simulink model "new_model"  (R2023a)
(part 4 of 4)

  Bus Selector:RadarSensor:4_OBJ_RCS_BS/5 -> RadarSensor:4.OBJ_RCS_5/1  "<OBJ_RCS_5>"
  Bus Selector:RadarSensor:4_OBJ_RCS_BS/6 -> RadarSensor:4.OBJ_RCS_6/1  "<OBJ_RCS_6>"
  Bus Selector:RadarSensor:4_OBJ_RCS_BS/7 -> RadarSensor:4.OBJ_RCS_7/1  "<OBJ_RCS_7>"
  Bus Selector:RadarSensor:4_OBJ_RCS_BS/8 -> RadarSensor:4.OBJ_RCS_8/1  "<OBJ_RCS_8>"
  Bus Selector:RadarSensor:4_OBJ_RCS_BS/9 -> RadarSensor:4.OBJ_RCS_9/1  "<OBJ_RCS_9>"
  Bus Selector:RadarSensor:4_OBJ_RCS_BS/10 -> RadarSensor:4.OBJ_RCS_10/1  "<OBJ_RCS_10>"
  Bus Selector:RadarSensor:4_OBJ_RCS_BS/11 -> RadarSensor:4.OBJ_RCS_11/1  "<OBJ_RCS_11>"
  Bus Selector:RadarSensor:4_OBJ_RCS_BS/12 -> RadarSensor:4.OBJ_RCS_12/1  "<OBJ_RCS_12>"
  Bus Selector:RadarSensor:4_OBJ_RCS_BS/13 -> RadarSensor:4.OBJ_RCS_13/1  "<OBJ_RCS_13>"
  Bus Selector:RadarSensor:4_OBJ_RCS_BS/14 -> RadarSensor:4.OBJ_RCS_14/1  "<OBJ_RCS_14>"
  Bus Selector:RadarSensor:4_OBJ_RCS_BS/15 -> RadarSensor:4.OBJ_RCS_15/1  "<OBJ_RCS_15>"
  Bus Selector:RadarSensor:4_OBJ_RCS_BS/16 -> RadarSensor:4.OBJ_RCS_16/1  "<OBJ_RCS_16>"
  Bus Selector:RadarSensor:4_OBJ_RCS_BS/17 -> RadarSensor:4.OBJ_RCS_17/1  "<OBJ_RCS_17>"
  Bus Selector:RadarSensor:4_OBJ_RCS_BS/18 -> RadarSensor:4.OBJ_RCS_18/1  "<OBJ_RCS_18>"
  Bus Selector:RadarSensor:4_OBJ_RCS_BS/19 -> RadarSensor:4.OBJ_RCS_19/1  "<OBJ_RCS_19>"
  Bus Selector:RadarSensor:4_OBJ_RCS_BS/20 -> RadarSensor:4.OBJ_RCS_20/1  "<OBJ_RCS_20>"
  Bus Selector:RadarSensor:4_OBJ_RCS_BS/21 -> RadarSensor:4.OBJ_RCS_21/1  "<OBJ_RCS_21>"
  Bus Selector:RadarSensor:4_OBJ_RCS_BS/22 -> RadarSensor:4.OBJ_RCS_22/1  "<OBJ_RCS_22>"
  Bus Selector:RadarSensor:4_OBJ_RCS_BS/23 -> RadarSensor:4.OBJ_RCS_23/1  "<OBJ_RCS_23>"
  Bus Selector:RadarSensor:4_OBJ_RCS_BS/24 -> RadarSensor:4.OBJ_RCS_24/1  "<OBJ_RCS_24>"
  Bus Selector:RadarSensor:4_OBJ_RCS_BS/25 -> RadarSensor:4.OBJ_RCS_25/1  "<OBJ_RCS_25>"
  Bus Selector:RadarSensor:4_OBJ_RCS_BS/26 -> RadarSensor:4.OBJ_RCS_26/1  "<OBJ_RCS_26>"
  Bus Selector:RadarSensor:4_OBJ_RCS_BS/27 -> RadarSensor:4.OBJ_RCS_27/1  "<OBJ_RCS_27>"
  Bus Selector:RadarSensor:4_OBJ_RCS_BS/28 -> RadarSensor:4.OBJ_RCS_28/1  "<OBJ_RCS_28>"
  Bus Selector:RadarSensor:4_OBJ_RCS_BS/29 -> RadarSensor:4.OBJ_RCS_29/1  "<OBJ_RCS_29>"
  Bus Selector:RadarSensor:4_OBJ_RCS_BS/30 -> RadarSensor:4.OBJ_RCS_30/1  "<OBJ_RCS_30>"
  Bus Selector:RadarSensor:4_OBJ_RCS_BS/31 -> RadarSensor:4.OBJ_RCS_31/1  "<OBJ_RCS_31>"
  Bus Selector:RadarSensor:4_OBJ_RCS_BS/32 -> RadarSensor:4.OBJ_RCS_32/1  "<OBJ_RCS_32>"
  Bus Selector:RadarSensor:4_OBJ_RCS_BS/33 -> RadarSensor:4.OBJ_RCS_33/1  "<OBJ_RCS_33>"
  Bus Selector:RadarSensor:4_OBJ_RCS_BS/34 -> RadarSensor:4.OBJ_RCS_34/1  "<OBJ_RCS_34>"
  Bus Selector:RadarSensor:4_OBJ_RCS_BS/35 -> RadarSensor:4.OBJ_RCS_35/1  "<OBJ_RCS_35>"
  Bus Selector:RadarSensor:4_OBJ_RCS_BS/36 -> RadarSensor:4.OBJ_RCS_36/1  "<OBJ_RCS_36>"
  Bus Selector:RadarSensor:4_OBJ_RCS_BS/37 -> RadarSensor:4.OBJ_RCS_37/1  "<OBJ_RCS_37>"
  Bus Selector:RadarSensor:4_OBJ_RCS_BS/38 -> RadarSensor:4.OBJ_RCS_38/1  "<OBJ_RCS_38>"
  Bus Selector:RadarSensor:4_OBJ_RCS_BS/39 -> RadarSensor:4.OBJ_RCS_39/1  "<OBJ_RCS_39>"
  Bus Selector:RadarSensor:4_OBJ_RCS_BS/40 -> RadarSensor:4.OBJ_RCS_40/1  "<OBJ_RCS_40>"
  Bus Selector:RadarSensor:4_OBJ_RCS_BS/41 -> RadarSensor:4.OBJ_RCS_41/1  "<OBJ_RCS_41>"
  Bus Selector:RadarSensor:4_OBJ_RCS_BS/42 -> RadarSensor:4.OBJ_RCS_42/1  "<OBJ_RCS_42>"
  Bus Selector:RadarSensor:4_OBJ_RCS_BS/43 -> RadarSensor:4.OBJ_RCS_43/1  "<OBJ_RCS_43>"
  Bus Selector:RadarSensor:4_OBJ_RCS_BS/44 -> RadarSensor:4.OBJ_RCS_44/1  "<OBJ_RCS_44>"
  Bus Selector:RadarSensor:4_OBJ_RCS_BS/45 -> RadarSensor:4.OBJ_RCS_45/1  "<OBJ_RCS_45>"
  Bus Selector:RadarSensor:4_OBJ_RCS_BS/46 -> RadarSensor:4.OBJ_RCS_46/1  "<OBJ_RCS_46>"
  Bus Selector:RadarSensor:4_OBJ_RCS_BS/47 -> RadarSensor:4.OBJ_RCS_47/1  "<OBJ_RCS_47>"
  Bus Selector:RadarSensor:4_OBJ_RCS_BS/48 -> RadarSensor:4.OBJ_RCS_48/1  "<OBJ_RCS_48>"
  Bus Selector:RadarSensor:4_OBJ_RCS_BS/49 -> RadarSensor:4.OBJ_RCS_49/1  "<OBJ_RCS_49>"
  Bus Selector:RadarSensor:4_OBJ_RCS_BS/50 -> RadarSensor:4.OBJ_RCS_50/1  "<OBJ_RCS_50>"
  Bus Selector:RadarSensor:4_OBJ_RCS_BS/51 -> RadarSensor:4.OBJ_RCS_51/1  "<OBJ_RCS_51>"
  Bus Selector:RadarSensor:4_OBJ_RCS_BS/52 -> RadarSensor:4.OBJ_RCS_52/1  "<OBJ_RCS_52>"
  Bus Selector:RadarSensor:4_OBJ_RCS_BS/53 -> RadarSensor:4.OBJ_RCS_53/1  "<OBJ_RCS_53>"
  Bus Selector:RadarSensor:4_OBJ_RCS_BS/54 -> RadarSensor:4.OBJ_RCS_54/1  "<OBJ_RCS_54>"
  Bus Selector:RadarSensor:4_OBJ_RCS_BS/55 -> RadarSensor:4.OBJ_RCS_55/1  "<OBJ_RCS_55>"
  Bus Selector:RadarSensor:4_OBJ_RCS_BS/56 -> RadarSensor:4.OBJ_RCS_56/1  "<OBJ_RCS_56>"
  Bus Selector:RadarSensor:4_OBJ_RCS_BS/57 -> RadarSensor:4.OBJ_RCS_57/1  "<OBJ_RCS_57>"
  Bus Selector:RadarSensor:4_OBJ_RCS_BS/58 -> RadarSensor:4.OBJ_RCS_58/1  "<OBJ_RCS_58>"
  Bus Selector:RadarSensor:4_OBJ_RCS_BS/59 -> RadarSensor:4.OBJ_RCS_59/1  "<OBJ_RCS_59>"
  Bus Selector:RadarSensor:4_OBJ_RCS_BS/60 -> RadarSensor:4.OBJ_RCS_60/1  "<OBJ_RCS_60>"
  Bus Selector:RadarSensor:4_OBJ_RCS_BS/61 -> RadarSensor:4.OBJ_RCS_61/1  "<OBJ_RCS_61>"
  Bus Selector:RadarSensor:4_OBJ_RCS_BS/62 -> RadarSensor:4.OBJ_RCS_62/1  "<OBJ_RCS_62>"
  Bus Selector:RadarSensor:4_OBJ_RCS_BS/63 -> RadarSensor:4.OBJ_RCS_63/1  "<OBJ_RCS_63>"
  Bus Selector:RadarSensor:4_OBJ_RCS_BS/64 -> RadarSensor:4.OBJ_RCS_64/1  "<OBJ_RCS_64>"
  Bus Selector:RadarSensor:4/1 -> RadarSensor:4.time/1  "<time>"
  Bus Selector:RadarSensor:4/2 -> RadarSensor:4.width/1  "<width>"
  Bus Selector:RadarSensor:4/3 -> RadarSensor:4.OBJ_ID/1, Bus Selector:RadarSensor:4_OBJ_ID_BS/1  "<OBJ_ID>"
  Bus Selector:RadarSensor:4/4 -> RadarSensor:4.OBJ_Class/1, Bus Selector:RadarSensor:4_OBJ_Class_BS/1  "<OBJ_Class>"
  Bus Selector:RadarSensor:4/5 -> RadarSensor:4.OBJ_S_Azimuth/1, Bus Selector:RadarSensor:4_OBJ_S_Azimuth_BS/1  "<OBJ_S_Azimuth>"
  Bus Selector:RadarSensor:4/6 -> RadarSensor:4.OBJ_S_Elevation/1, Bus Selector:RadarSensor:4_OBJ_S_Elevation_BS/1  "<OBJ_S_Elevation>"
  Bus Selector:RadarSensor:4/7 -> RadarSensor:4.OBJ_S_Velocity/1, Bus Selector:RadarSensor:4_OBJ_S_Velocity_BS/1  "<OBJ_S_Velocity>"
  Bus Selector:RadarSensor:4/8 -> RadarSensor:4.OBJ_S_Range/1, Bus Selector:RadarSensor:4_OBJ_S_Range_BS/1  "<OBJ_S_Range>"
  Bus Selector:RadarSensor:4/9 -> RadarSensor:4.OBJ_RCS/1, Bus Selector:RadarSensor:4_OBJ_RCS_BS/1  "<OBJ_RCS>"
  Bus Selector:UltrasonicSensor:0/1 -> UltrasonicSensor:0.time/1  "<time>"
  Bus Selector:UltrasonicSensor:0/2 -> UltrasonicSensor:0.width/1  "<width>"
  Bus Selector:UltrasonicSensor:0/3 -> UltrasonicSensor:0.distance/1  "<distance>"
  Bus Selector:UltrasonicSensor:1/1 -> UltrasonicSensor:1.time/1  "<time>"
  Bus Selector:UltrasonicSensor:1/2 -> UltrasonicSensor:1.width/1  "<width>"
  Bus Selector:UltrasonicSensor:1/3 -> UltrasonicSensor:1.distance/1  "<distance>"
  Bus Selector:UltrasonicSensor:2/1 -> UltrasonicSensor:2.time/1  "<time>"
  Bus Selector:UltrasonicSensor:2/2 -> UltrasonicSensor:2.width/1  "<width>"
  Bus Selector:UltrasonicSensor:2/3 -> UltrasonicSensor:2.distance/1  "<distance>"
  Bus Selector:UltrasonicSensor:3/1 -> UltrasonicSensor:3.time/1  "<time>"
  Bus Selector:UltrasonicSensor:3/2 -> UltrasonicSensor:3.width/1  "<width>"
  Bus Selector:UltrasonicSensor:3/3 -> UltrasonicSensor:3.distance/1  "<distance>"
  Bus Selector:UltrasonicSensor:4/1 -> UltrasonicSensor:4.time/1  "<time>"
  Bus Selector:UltrasonicSensor:4/2 -> UltrasonicSensor:4.width/1  "<width>"
  Bus Selector:UltrasonicSensor:4/3 -> UltrasonicSensor:4.distance/1  "<distance>"
  Bus Selector:UltrasonicSensor:5/1 -> UltrasonicSensor:5.time/1  "<time>"
  Bus Selector:UltrasonicSensor:5/2 -> UltrasonicSensor:5.width/1  "<width>"
  Bus Selector:UltrasonicSensor:5/3 -> UltrasonicSensor:5.distance/1  "<distance>"
  Bus Selector:UltrasonicSensor:6/1 -> UltrasonicSensor:6.time/1  "<time>"
  Bus Selector:UltrasonicSensor:6/2 -> UltrasonicSensor:6.width/1  "<width>"
  Bus Selector:UltrasonicSensor:6/3 -> UltrasonicSensor:6.distance/1  "<distance>"
  Bus Selector:UltrasonicSensor:7/1 -> UltrasonicSensor:7.time/1  "<time>"
  Bus Selector:UltrasonicSensor:7/2 -> UltrasonicSensor:7.width/1  "<width>"
  Bus Selector:UltrasonicSensor:7/3 -> UltrasonicSensor:7.distance/1  "<distance>"
  Bus Selector:UltrasonicSensor:8/1 -> UltrasonicSensor:8.time/1  "<time>"
  Bus Selector:UltrasonicSensor:8/2 -> UltrasonicSensor:8.width/1  "<width>"
  Bus Selector:UltrasonicSensor:8/3 -> UltrasonicSensor:8.distance/1  "<distance>"
  Bus Selector:UltrasonicSensor:9/1 -> UltrasonicSensor:9.time/1  "<time>"
  Bus Selector:UltrasonicSensor:9/2 -> UltrasonicSensor:9.width/1  "<width>"
  Bus Selector:UltrasonicSensor:9/3 -> UltrasonicSensor:9.distance/1  "<distance>"
  Bus Selector:UltrasonicSensor:10/1 -> UltrasonicSensor:10.time/1  "<time>"
  Bus Selector:UltrasonicSensor:10/2 -> UltrasonicSensor:10.width/1  "<width>"
  Bus Selector:UltrasonicSensor:10/3 -> UltrasonicSensor:10.distance/1  "<distance>"
  Bus Selector:UltrasonicSensor:11/1 -> UltrasonicSensor:11.time/1  "<time>"
  Bus Selector:UltrasonicSensor:11/2 -> UltrasonicSensor:11.width/1  "<width>"
  Bus Selector:UltrasonicSensor:11/3 -> UltrasonicSensor:11.distance/1  "<distance>"
  Bus Selector:GNSS:0/1 -> GNSS:0.Timestamp/1  "<Timestamp>"
  Bus Selector:GNSS:0/2 -> GNSS:0.Longitude/1  "<Longitude>"
  Bus Selector:GNSS:0/3 -> GNSS:0.Latitude/1  "<Latitude>"
  Bus Selector:GNSS:0/4 -> GNSS:0.Altitude/1  "<Altitude>"
  Bus Selector:GNSS:0/5 -> GNSS:0.Heading/1  "<Heading>"
  Bus Selector:GNSS:0/6 -> GNSS:0.Velocity/1  "<Velocity>"
  Bus Selector:IMU:0/1 -> IMU:0.Timestamp/1  "<Timestamp>"
  Bus Selector:IMU:0/2 -> IMU:0.ACC_X/1  "<ACC_X>"
  Bus Selector:IMU:0/3 -> IMU:0.ACC_Y/1  "<ACC_Y>"
  Bus Selector:IMU:0/4 -> IMU:0.ACC_Z/1  "<ACC_Z>"
  Bus Selector:IMU:0/5 -> IMU:0.Gyro_X/1  "<Gyro_X>"
  Bus Selector:IMU:0/6 -> IMU:0.Gyro_Y/1  "<Gyro_Y>"
  Bus Selector:IMU:0/7 -> IMU:0.Gyro_Z/1  "<Gyro_Z>"
  Bus Selector:IMU:0/8 -> IMU:0.Yaw/1  "<Yaw>"
  Bus Selector:IMU:0/9 -> IMU:0.Pitch/1  "<Pitch>"
  Bus Selector:IMU:0/10 -> IMU:0.Roll/1  "<Roll>"
